simulink model "Pendulum_Sim_Model"  (R2019b)
settings: Solver=VariableStepAuto  StartTime=0.0  StopTime=20  RelTol=1e-3
values from neighbouring files (symbols this model uses):
  b = 0.03    [Robot_Model_Param_Pend.m]
  g = 9.8    [Robot_Model_Param_Pend.m]
  l = 0.31    [Robot_Model_Param_Pend.m]
  m = 0.3    [Robot_Model_Param_Pend.m]
undefined symbols (not defined in the file or in its folder): CPden, CPnum
settings Model: Creator=aclang  LastModifiedBy=ZYT

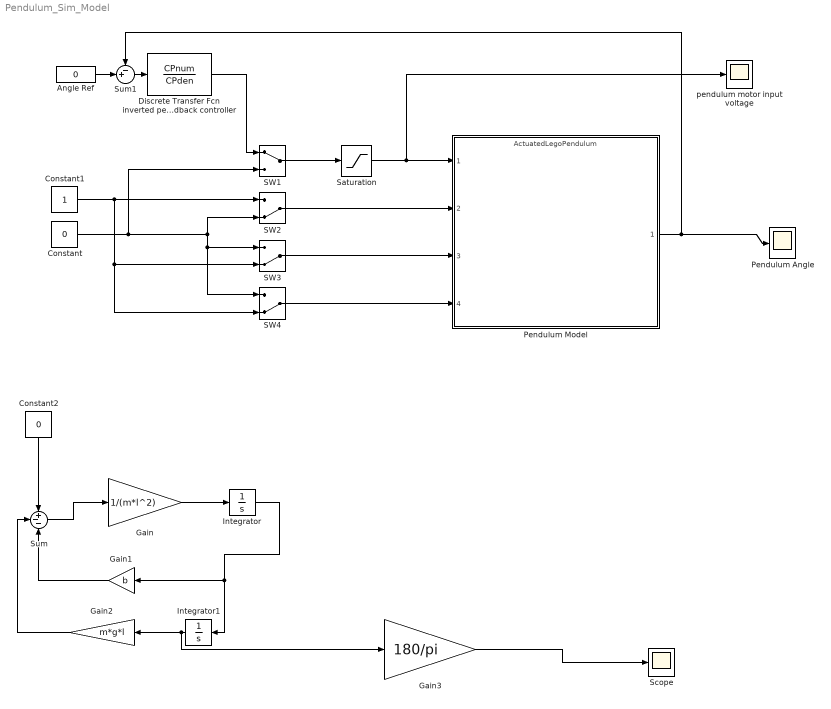
== system Pendulum_Sim_Model ==
  "  Saturation" : Saturate  UpperLimit=100  LowerLimit=-100
  Angle Ref : Constant  Value=0
  Constant : Constant  Value=0
  Constant1 : Constant
  Constant2 : Constant  Value=0
  Discrete Transfer Fcn inverted pendulum feedback controller : DiscreteTransferFcn  Numerator=CPnum  Denominator=CPden
  Gain : Gain  Gain=1/(m*l^2)
  Gain1 : Gain  Gain=b
  Gain2 : Gain  Gain=m*g*l
  Gain3 : Gain  Gain=180/pi
  Integrator : Integrator
  Integrator1 : Integrator  InitialCondition=pi/2
  Pendulum Angle : Scope
  Pendulum Model : ModelReference  StopFcn=|  ModelNameDialog=ActuatedLegoPendulum.slxp  ModelReferenceVersion=1.55  CopyOfModelProtected=on
      | %%%%%%%%%%%%%%%%%%%%%%%%%%%%%%%%%%%%%%%%%%%%%%%%%%%%%%%%%%%%%%%%%%%%%%%%%%
      | % Script for producing pendulum animation from data 
      | % generated by Simulink model Pendulum_Sim_Model
      | %
      | %%%%%%%%%%%%%%%%%%%%%%%%%%%%%%%%%%%%%%%%%%%%%%%%%%%%%%%%%%%%%%%%%%%%%%%%%%
      | % Created by M.Cantoni on 2020-10-06
      | %
      | % Updated by Armaghan Zafar on 2021-09-21
      | % to run with Workshop 4 design by Adair Lang
      | %%%%%%%%%%%%%%%%%%%%%%%%%%%%%%%%%%%%%%%%%%%%%%%%%%%%%%%%%%%%%%%%%%%%%%%%%
      | 
      | %%%% sim_ini is the pendulum XY data
      | 
      | sim_ini_dt = max(out.sim_ini.time)/50;   %% Reduces total no. of point to plot
      | sim_ini_loops = round(max(out.sim_ini.time)/sim_ini_dt);
      | 
      | sim_ini_xpend = [];
      | sim_ini_ypend = [];
      | 
      | for sim_ini_i = 1:sim_ini_loops
      |     sim_ini_ind = find(out.sim_ini.time <= (sim_ini_i-1)*sim_ini_dt);
      |     sim_ini_xpend = [sim_ini_xpend out.sim_ini.data(max(sim_ini_ind),1)];
      |     sim_ini_ypend = [sim_ini_ypend out.sim_ini.data(max(sim_ini_ind),2)];
      | end
      | 
      | sim_ini_xmax = 1.5*max(abs(sim_ini_xpend));
      | sim_ini_xmin = -sim_ini_xmax;
      | 
      | sim_ini_ymax = 1.5*max(abs(sim_ini_ypend));
      | sim_ini_ymin = -sim_ini_ymax;
      | 
      | figure;
      | plot(sim_ini_xmin,sim_ini_ymin,sim_ini_xmax,sim_ini_ymax);
      | xlabel('Position of Pendulum');
      | ylabel('Position above/below the pivot');
      | title('Pendulum (circle) on a pivot (square)');
      | axis tight manual
      | sim_ini_ax = gca;
      | sim_ini_ax.NextPlot = 'replaceChildren';
      | 
      | set(gca,'visible','off')
      | sim_ini_fig = gcf;
      | sim_ini_fig.MenuBar = 'none';
      | 
      | for sim_ini_i = 1:sim_ini_loops %length(out.sim_ini.time)
      |     plot(0,sim_ini_xpend(1),'ks',sim_ini_xpend(sim_ini_i),sim_ini_ypend(sim_ini_i),'bo',[0,sim_ini_xpend(sim_ini_i)],[sim_ini_xpend(1),sim_ini_ypend(sim_ini_i)],'k-','LineWidth',2,'MarkerSize',12);
      |     set(gca,'visible','off')
      |     sim_ini_fig = gcf;
      |     sim_ini_fig.MenuBar = 'none';
      |     drawnow
      | end
      | 
      | out.sim_ini = [];
      | close (sim_ini_fig);
      | clear sim_ini_*
  SW1 : ManualSwitch
  "SW2 " : ManualSwitch  CurrentSetting=0
  SW3 : ManualSwitch  CurrentSetting=0
  SW4 : ManualSwitch  CurrentSetting=0
  Scope : Scope
  Sum : Sum  Inputs=+--
  Sum1 : Sum  Inputs=-+|
  pendulum motor input voltage : Scope
  wires:
  Constant1/1 -> SW4/2, SW3/2, "SW2 "/1
  Constant/1 -> SW1/2, SW3/1, SW4/1, "SW2 "/2
  "SW2 "/1 -> Pendulum Model/2
  SW3/1 -> Pendulum Model/3
  SW4/1 -> Pendulum Model/4
  Discrete Transfer Fcn inverted pendulum feedback controller/1 -> SW1/1
  SW1/1 -> "  Saturation"/1
  "  Saturation"/1 -> pendulum motor input voltage/1, Pendulum Model/1
  Sum1/1 -> Discrete Transfer Fcn inverted pendulum feedback controller/1
  Angle Ref/1 -> Sum1/2
  Pendulum Model/1 -> Sum1/1, Pendulum Angle/1
  Constant2/1 -> Sum/1
  Gain/1 -> Integrator/1
  Integrator/1 -> Integrator1/1, Gain1/1
  Integrator1/1 -> Gain3/1, Gain2/1
  Gain1/1 -> Sum/3
  Gain2/1 -> Sum/2
  Sum/1 -> Gain/1
  Gain3/1 -> Scope/1
